simulink model "Marine_LocoMotive_UAV"  (R2018a)
settings: Solver=ode4  StartTime=0.0  StopTime=60  FixedStep=T  RelTol=1e-3
values from neighbouring files (symbols this model uses):
  a_11 = 0.05*m_b    (= 0.625)    [Marine_LocoMotive_UAV_parameters.m]
  a_33 = m_b    (= 12.5)    [Marine_LocoMotive_UAV_parameters.m]
  A_w = 1*1.5/2    (= 0.75)    [Marine_LocoMotive_UAV_parameters.m]
  A_w2 = 1*0.27/2    (= 0.135)    [Marine_LocoMotive_UAV_parameters.m]
  alpha_bar = pi/4    (= 0.785398163397)    [Marine_LocoMotive_UAV_parameters.m]
  Am = sysd.denominator{1}    [Marine_LocoMotive_UAV_parameters.m]
  Am1_LPF = sysd.denominator{1}    [Marine_LocoMotive_UAV_parameters.m]
  Am2_LPF = sysd.denominator{1}    [Marine_LocoMotive_UAV_parameters.m]
  AmAlpha_LPF = sysd.denominator{1}    [Marine_LocoMotive_UAV_parameters.m]
  AmV_LPF = sysd.denominator{1}    [Marine_LocoMotive_UAV_parameters.m]
  AmZ_LPF = sysd.denominator{1}    [Marine_LocoMotive_UAV_parameters.m]
  b_11 = 0    [Marine_LocoMotive_UAV_parameters.m]
  b_33 = 2*m_b*omega_h    (= 27.5578302946)    [Marine_LocoMotive_UAV_parameters.m]
  Bm = sysd.numerator{1}    [Marine_LocoMotive_UAV_parameters.m]
  Bm1_LPF = sysd.numerator{1}    [Marine_LocoMotive_UAV_parameters.m]
  Bm2_LPF = sysd.numerator{1}    [Marine_LocoMotive_UAV_parameters.m]
  BmAlpha_LPF = sysd.numerator{1}    [Marine_LocoMotive_UAV_parameters.m]
  BmV_LPF = sysd.numerator{1}    [Marine_LocoMotive_UAV_parameters.m]
  BmZ_LPF = sysd.numerator{1}    [Marine_LocoMotive_UAV_parameters.m]
  C_S = [5;9]*10^-3    [Marine_LocoMotive_UAV_parameters.m]
  D_x = b_11 + D_s(1)    [Marine_LocoMotive_UAV_parameters.m]
  D_z = b_33 + D_s(2)    [Marine_LocoMotive_UAV_parameters.m]
  dc_M_p = 6.7    [Marine_LocoMotive_UAV_parameters.m]
  Delta_h = (A_im/A_b-0.5)*h_b    (= -0.0625)    [Marine_LocoMotive_UAV_parameters.m]
  epsilon_1 = 5    [Marine_LocoMotive_UAV_parameters.m]
  epsilon_w = 0    [Marine_LocoMotive_UAV_parameters.m]
  epsilon_w2 = pi    (= 3.14159265359)    [Marine_LocoMotive_UAV_parameters.m]
  g = 9.81    [Marine_LocoMotive_UAV_parameters.m]
  gamma_d_p = 2*0.3/0.03*2*0.2*12/4    (= 24)    [Marine_LocoMotive_UAV_parameters.m]
  H = 10    [Marine_LocoMotive_UAV_parameters.m]
  h_b = 0.25    [Marine_LocoMotive_UAV_parameters.m]
  J_a = m_u*Lc_0^2 + (m_u*(Lc_0/2)^2+m_u*Lc_0/12)    (= 111.3)    [Marine_LocoMotive_UAV_parameters.m]
  J_b = m_b*h_b*l_b/12    (= 0.208333333333)    [Marine_LocoMotive_UAV_parameters.m]
  J_u = 0.03    [Marine_LocoMotive_UAV_parameters.m]
  K = 20    [Marine_LocoMotive_UAV_parameters.m]
  k3 = 4.5    [Marine_LocoMotive_UAV_parameters.m]
  k4 = 2    [Marine_LocoMotive_UAV_parameters.m]
  k_w = omega_w^2/g    (= 0.123862835563)    [Marine_LocoMotive_UAV_parameters.m]
  k_w2 = omega_w2^2/g    (= 0.447144836384)    [Marine_LocoMotive_UAV_parameters.m]
  kd_a = 7    [Marine_LocoMotive_UAV_parameters.m]
  kd_t = 6    [Marine_LocoMotive_UAV_parameters.m]
  kd_T = 0.3    [Marine_LocoMotive_UAV_parameters.m]
  kd_x = 5    [Marine_LocoMotive_UAV_parameters.m]
  kd_z = 2    [Marine_LocoMotive_UAV_parameters.m]
  ki_a = 2    [Marine_LocoMotive_UAV_parameters.m]
  ki_T = 0.8    [Marine_LocoMotive_UAV_parameters.m]
  ki_x = 1.2    [Marine_LocoMotive_UAV_parameters.m]
  ki_z = 1    [Marine_LocoMotive_UAV_parameters.m]
  kp_a = 7    [Marine_LocoMotive_UAV_parameters.m]
  kp_t = 10    [Marine_LocoMotive_UAV_parameters.m]
  kp_T = 5    [Marine_LocoMotive_UAV_parameters.m]
  kp_x = 7    [Marine_LocoMotive_UAV_parameters.m]
  kp_z = 3    [Marine_LocoMotive_UAV_parameters.m]
  L = 0.2    [Marine_LocoMotive_UAV_parameters.m]
  l_b = 0.8    [Marine_LocoMotive_UAV_parameters.m]
  Lc_0 = 7    [Marine_LocoMotive_UAV_parameters.m]
  LIMIT_CMD_PITCH = 45*pi/180    (= 0.785398163397)    [Marine_LocoMotive_UAV_parameters.m]
  LIMIT_uCMD_HEIGHT = 3.5*K    (= 70)    [Marine_LocoMotive_UAV_parameters.m]
  M_a = m_u*Lc_0 + m_c*Lc_0    (= 16.1)    [Marine_LocoMotive_UAV_parameters.m]
  m_b = rho_w*Vol_b/4    (= 12.5)    [Marine_LocoMotive_UAV_parameters.m]
  m_c = 0.5    [Marine_LocoMotive_UAV_parameters.m]
  m_u = 1.8    [Marine_LocoMotive_UAV_parameters.m]
  nu_w = 1.787*10^-6    (= 1.787e-06)    [Marine_LocoMotive_UAV_parameters.m]
  omega_w = 2*pi/T_w    (= 1.10231321179)    [Marine_LocoMotive_UAV_parameters.m]
  omega_w2 = 2*pi/T_w2    (= 2.09439510239)    [Marine_LocoMotive_UAV_parameters.m]
  rho_w = 1000    [Marine_LocoMotive_UAV_parameters.m]
  T = 1/100    (= 0.01)    [Marine_LocoMotive_UAV_parameters.m]
  Theta0 = atan2(V_bar*D_x*cos(alpha_bar_0),V_bar*D_x*sin(alpha_bar_0)+m_u*g*cos(alpha_bar_0))    [Marine_LocoMotive_UAV_parameters.m]
  u_s = w_dir*A_w^2*omega_w*k_w*exp(2*k_w*(-Delta_h/2))    [Marine_LocoMotive_UAV_parameters.m]
  u_s2 = w_dir2*A_w2^2*omega_w2*k_w2*exp(2*k_w2*(-Delta_h/2))    [Marine_LocoMotive_UAV_parameters.m]
  u_t = 0*0.2*1    (= 0)    [Marine_LocoMotive_UAV_parameters.m]
  u_w = 0*0.2    (= 0)    [Marine_LocoMotive_UAV_parameters.m]
  V0_b = [u_t+u_w+u_s+u_s2+v_x_w, v_z_w]    [Marine_LocoMotive_UAV_parameters.m]
  V_bar = 5    [Marine_LocoMotive_UAV_parameters.m]
  Vol_b = A_b*l_b    (= 0.05)    [Marine_LocoMotive_UAV_parameters.m]
  w_dir = 1    [Marine_LocoMotive_UAV_parameters.m]
  w_dir2 = 1    [Marine_LocoMotive_UAV_parameters.m]
  X0_b = [0,H+Zeta_0-Delta_h]    [Marine_LocoMotive_UAV_parameters.m]
  zu_bar = X0_b(2) + Lc_0*sin(alpha_bar_0)    [Marine_LocoMotive_UAV_parameters.m]
undefined symbols (not defined in the file or in its folder): DiscIntNeverNeededParam, k_Da, k_Pa, R_b, Zg
libraries: simulink x30, simulink_extras x3
(part 3 of 3)

== system Marine_LocoMotive_UAV/UAV control/u_alpha1 ==
  note: PID
  alpha : Inport
  Xb_ddot1 : Inport  Port=2
  alpha_ref : Inport  Port=3
  "alpha_dot " : Inport  Port=4
  " alpha" : InportShadow
  Add3 : Sum  Inputs=+--
  Add4 : Sum  Inputs=3
  Discrete Transfer Fcn : DiscreteTransferFcn  Commented=on  Numerator=BmAlpha_LPF  Denominator=AmAlpha_LPF
  Discrete Derivative2 : simulink/Discrete/Discrete Derivative  gainval=1.0  ICPrevScaledInput=alpha_bar/T  OutMin=[]  OutMax=[]  OutDataType=fixdt(1, 16)  OutScaling=2^-10  DoSatur=off
  Discrete-Time Integrator : DiscreteIntegrator  SampleTime=-1  LimitOutput=on  UpperSaturationLimit=1  LowerSaturationLimit=-1  ICPrevOutput=DiscIntNeverNeededParam  ICPrevScaledInput=DiscIntNeverNeededParam
  Gain10 : Gain  Gain=kd_a*2
  Gain12 : Gain  Gain=Lc_0
  Gain15 : Gain  Gain=Lc_0
  Gain4 : Gain  Gain=m_u
  Gain6 : Gain  Gain=g
  Gain8 : Gain  Gain=kp_a
  Gain9 : Gain  Gain=ki_a*2
  IC : InitialCondition  Value=0
  Mux : Mux  Inputs=2
  Mux1 : Mux
  Product2 : Product
  Product4 : Product
  Scope{10..11,17..18,26} (5 alike) : Scope
  Sum1 : Sum  Inputs=|+-
  Sum2 : Sum  Inputs=|+-
  Sum7 : Sum  Inputs=|+-
  Trigonometric Function2 : Trigonometry  Operator=cos
  Trigonometric Function3 : Trigonometry  Operator=sincos
  "alpha " : InportShadow
  pid_fb : Scope
  tuner : Gain  Gain=2
  "ua_fb " : Scope
  very high frequency not useful : Gain
  xb_ddot 1 : Selector  InputPortWidth=2  IndexOptions=Index vector (dialog)  Indices=1  OutputSizes=1
  zb_ddot2 : Selector  InputPortWidth=2  IndexOptions=Index vector (dialog)  Indices=1  OutputSizes=1
  u_a : Outport
  wires:
  Gain12/1 -> tuner/1
  very high frequency not useful/1 -> Add3/2
  Mux1/1 -> pid_fb/1
  alpha/1 -> Trigonometric Function2/1
  "alpha "/1 -> Trigonometric Function3/1
  " alpha"/1 -> Sum2/1
  Mux/1 -> Scope26/1
  Trigonometric Function3/2 -> Product4/2
  Discrete-Time Integrator/1 -> Add4/2, Mux1/2  "i"
  Gain15/1 -> very high frequency not useful/1, Scope11/1
  Trigonometric Function2/1 -> Gain6/1
  Trigonometric Function3/1 -> Product2/2
  Product2/1 -> Sum7/1
  Gain9/1 -> Discrete-Time Integrator/1
  xb_ddot 1/1 -> Product2/1
  Gain10/1 -> Mux/2, Mux/1, Add4/3, Mux1/3  "d"
  Xb_ddot1/1 -> xb_ddot 1/1, zb_ddot2/1
  Discrete Derivative2/1 -> IC/1
  Add3/1 -> Gain4/1
  Gain8/1 -> Add4/1, Mux1/1  "p"
  zb_ddot2/1 -> Product4/1
  Product4/1 -> Sum7/2
  tuner/1 -> Add3/3, "ua_fb "/1
  Gain4/1 -> u_a/1  "u_a"
  "alpha_dot "/1 -> Sum1/1
  Add4/1 -> Gain12/1, Mux1/4  "fb"
  alpha_ref/1 -> Discrete Derivative2/1, Sum2/2, Scope18/1
  Sum1/1 -> Gain10/1
  Sum2/1 -> Gain8/1, Gain9/1
  Sum7/1 -> Gain15/1
  Gain6/1 -> Add3/1, Scope10/1
  IC/1 -> Sum1/2, Scope17/1

== system Marine_LocoMotive_UAV/Quadrotor+buoy/3-DOF equations of motion Earth frame/C_123 ==
  "alpha " : Inport
  alpha_dot : Inport  Port=2
  Constant : Constant  Value=0
  Gain : Gain  Gain=-M_a
  Gain1 : Gain  Gain=-M_a
  Product : Product
  Product1 : Product
  Signal Specification1 : SignalSpecification  Dimensions=3
  Signal Specification2 : SignalSpecification  Dimensions=3
  Signal Specification3 : SignalSpecification  Dimensions=3
  Trigonometric Function : Trigonometry  Operator=sincos
  Vector Concatenate1 : Concatenate  NumInputs=3  Mode=Multidimensional array  ConcatenateDimension=2
  Vector Concatenate2 : Concatenate  NumInputs=3
  Vector Concatenate3 : Concatenate  NumInputs=3
  Vector Concatenate4 : Concatenate  NumInputs=3
  C_123 : Outport
  wires:
  Signal Specification3/1 -> Vector Concatenate1/3
  Signal Specification2/1 -> Vector Concatenate1/2
  Signal Specification1/1 -> Vector Concatenate1/1
  Vector Concatenate1/1 -> C_123/1
  Trigonometric Function/2 -> Gain1/1
  Trigonometric Function/1 -> Gain/1
  "alpha "/1 -> Trigonometric Function/1
  Vector Concatenate4/1 -> Signal Specification2/1
  Vector Concatenate2/1 -> Signal Specification1/1
  Vector Concatenate3/1 -> Signal Specification3/1
  Gain/1 -> Product/1
  Gain1/1 -> Product1/1
  Product1/1 -> Vector Concatenate3/1
  Product/1 -> Vector Concatenate3/2
  alpha_dot/1 -> Product1/2, Product/2
  Constant/1 -> Vector Concatenate3/3, Vector Concatenate4/3, Vector Concatenate4/2, Vector Concatenate4/1, Vector Concatenate2/3, Vector Concatenate2/2, Vector Concatenate2/1

== system Marine_LocoMotive_UAV/Quadrotor+buoy/3-DOF equations of motion Earth frame/D_123 ==
  eta_dot_tilde : Inport
  theta_b : Inport  Port=2
  dh : Inport  Port=3
  Constant6 : Constant  Value=[0 0 0]
  Constant7 : Constant  Value=0
  Scope : Scope
  Scope1 : Scope
  Scope2 : Scope
  Vector Concatenate1 : Concatenate  NumInputs=3  Mode=Multidimensional array  ConcatenateDimension=2
  Vector Concatenate2 : Concatenate  NumInputs=3
  Vector Concatenate3 : Concatenate  NumInputs=3
  Vector Concatenate4 : Concatenate
  Vector Concatenate5 : Concatenate
  Vector Concatenate6 : Concatenate
  Water Daming : Subsystem
  Water Daming1 : Subsystem
  D_123 : Outport
  wires:
  Water Daming/2(D22_I) -> Vector Concatenate3/2, Vector Concatenate5/2
  Constant7/1 -> Vector Concatenate3/3, Vector Concatenate2/3
  Constant6/1 -> Vector Concatenate1/3
  Vector Concatenate2/1 -> Vector Concatenate1/1
  Water Daming/1(D11_I) -> Vector Concatenate4/2, Vector Concatenate2/1
  Vector Concatenate3/1 -> Vector Concatenate1/2
  theta_b/1 -> Water Daming1/1(theta), Water Daming/1(theta_b)
  eta_dot_tilde/1 -> Water Daming/2(eta_dot_tilde)
  dh/1 -> Water Daming/3(dh)
  Vector Concatenate1/1 -> D_123/1
  Vector Concatenate4/1 -> Scope/1
  Water Daming1/1(D11_I) -> Vector Concatenate4/1
  Vector Concatenate5/1 -> Scope1/1
  Water Daming1/2(D22_I) -> Vector Concatenate5/1
  Vector Concatenate6/1 -> Scope2/1
  Water Daming1/3(D12_I) -> Vector Concatenate6/1
  Water Daming/3(D12_I) -> Vector Concatenate3/1, Vector Concatenate6/2, Vector Concatenate2/2

== system Marine_LocoMotive_UAV/Quadrotor+buoy/3-DOF equations of motion Earth frame/FB ==
  Constant1 : Constant  Value=rho_w*g
  F_B : Product
  Out1 : Outport
  wires:
  F_B/1 -> Out1/1
  [Vol_im] -> F_B/1
  Constant1/1 -> F_B/2

== system Marine_LocoMotive_UAV/Quadrotor+buoy/3-DOF equations of motion Earth frame/G1 ==
  Constant3 : Constant  Value=0
  Constant4 : Constant  Value=(m_b)*g
  Vector Concatenate : Concatenate
  G : Outport
  wires:
  Vector Concatenate/1 -> G/1
  Constant3/1 -> Vector Concatenate/1  "u1"
  Constant4/1 -> Vector Concatenate/2  "u2"

== system Marine_LocoMotive_UAV/Quadrotor+buoy/3-DOF equations of motion Earth frame/G123 ==
  alpha : Inport
  Constant3 : Constant  Value=0
  Constant4 : Constant  Value=(m_b+m_u+m_c)*g
  Constant5 : Constant  Value=m_u*g*L
  Product5 : Product  Inputs=**  SaturateOnIntegerOverflow=on  InputSameDT=on  OutDataTypeStr=Inherit: Same as first input
  Trigonometric Function : Trigonometry  Operator=cos
  Vector Concatenate : Concatenate  NumInputs=3
  G : Outport
  wires:
  Constant5/1 -> Product5/1
  Trigonometric Function/1 -> Product5/2
  Product5/1 -> Vector Concatenate/3  "u3"
  Constant4/1 -> Vector Concatenate/2  "u2"
  Constant3/1 -> Vector Concatenate/1  "u1"
  alpha/1 -> Trigonometric Function/1
  Vector Concatenate/1 -> G/1

== system Marine_LocoMotive_UAV/Quadrotor+buoy/3-DOF equations of motion Earth frame/M_12 ==
  theta : Inport
  Bias : Bias
  Bias1 : Bias
  Signal Specification1 : SignalSpecification  Dimensions=2
  Signal Specification2 : SignalSpecification  Dimensions=2
  Vector Concatenate1 : Concatenate  Mode=Multidimensional array  ConcatenateDimension=2
  Vector Concatenate2 : Concatenate
  Vector Concatenate3 : Concatenate
  added mass : Subsystem
  M_12 : Outport
  wires:
  Signal Specification2/1 -> Vector Concatenate1/2
  Signal Specification1/1 -> Vector Concatenate1/1
  Vector Concatenate1/1 -> M_12/1
  Bias1/1 -> Vector Concatenate3/2
  Bias/1 -> Vector Concatenate2/1
  added mass/2(M22_I) -> Bias1/1
  added mass/3(M12_I) -> Vector Concatenate2/2, Vector Concatenate3/1
  Vector Concatenate2/1 -> Signal Specification1/1
  added mass/1(M11_I) -> Bias/1
  Vector Concatenate3/1 -> Signal Specification2/1
  theta/1 -> added mass/1(theta)

== system Marine_LocoMotive_UAV/Quadrotor+buoy/3-DOF equations of motion Earth frame/M_123 ==
  theta : Inport
  alpha : Inport  Port=2
  Bias : Bias  Bias=m_u+m_c
  Bias1 : Bias  Bias=m_u+m_c
  Buoy Inertia : Subsystem
  Constant : Constant  Value=J_a
  Gain : Gain  Gain=-M_a
  Gain1 : Gain  Gain=M_a
  Signal Specification1 : SignalSpecification  Dimensions=3
  Signal Specification2 : SignalSpecification  Dimensions=3
  Signal Specification3 : SignalSpecification  Dimensions=3
  Trigonometric Function : Trigonometry  Operator=sincos
  Vector Concatenate1 : Concatenate  NumInputs=3  Mode=Multidimensional array  ConcatenateDimension=2
  Vector Concatenate2 : Concatenate  NumInputs=3
  Vector Concatenate3 : Concatenate  NumInputs=3
  Vector Concatenate4 : Concatenate  NumInputs=3
  M_123 : Outport
  wires:
  theta/1 -> Buoy Inertia/1(theta)
  Vector Concatenate3/1 -> Signal Specification2/1
  Buoy Inertia/1(M11_I) -> Bias/1
  Vector Concatenate2/1 -> Signal Specification1/1
  Vector Concatenate4/1 -> Signal Specification3/1
  Buoy Inertia/3(M12_I) -> Vector Concatenate2/2, Vector Concatenate3/1
  Gain/1 -> Vector Concatenate2/3, Vector Concatenate4/1
  Buoy Inertia/2(M22_I) -> Bias1/1
  Bias/1 -> Vector Concatenate2/1
  Bias1/1 -> Vector Concatenate3/2
  alpha/1 -> Trigonometric Function/1
  Trigonometric Function/1 -> Gain/1
  Trigonometric Function/2 -> Gain1/1
  Gain1/1 -> Vector Concatenate4/2, Vector Concatenate3/3
  Constant/1 -> Vector Concatenate4/3
  Vector Concatenate1/1 -> M_123/1
  Signal Specification1/1 -> Vector Concatenate1/1
  Signal Specification2/1 -> Vector Concatenate1/2
  Signal Specification3/1 -> Vector Concatenate1/3

== system Marine_LocoMotive_UAV/Quadrotor+buoy/3-DOF equations of motion Earth frame/Tension from Buoy, X direction ==
  alpha : Inport
  M12 : Inport  Port=2
  D12 : Inport  Port=3
  Vr,Wr : Inport  Port=4
  Xb_ddot : Inport  Port=5
  G : Inport  Port=6
  FB : Inport  Port=7
  Add1 : Sum  Inputs=+++-
  Constant : Constant  Value=0
  Math Function : Math  Operator=reciprocal  SaturateOnIntegerOverflow=on
  Math Function1 : Math  Operator=reciprocal  SaturateOnIntegerOverflow=on
  Product1 : Product
  Product2 : Product  Inputs=**  Multiplication=Matrix(*)
  Product3 : Product  Inputs=**  Multiplication=Matrix(*)
  Scope5 : Scope
  Trigonometric Function3 : Trigonometry  Operator=sincos
  Vector Concatenate2 : Concatenate
  Vector Concatenate3 : Concatenate
  T x,z : Outport
  wires:
  alpha/1 -> Trigonometric Function3/1
  M12/1 -> Product2/1
  Vr,Wr/1 -> Product3/2
  D12/1 -> Product3/1
  Xb_ddot/1 -> Product2/2
  G/1 -> Add1/3
  Product2/1 -> Add1/2
  Trigonometric Function3/2 -> Math Function/1
  Trigonometric Function3/1 -> Math Function1/1
  Product3/1 -> Add1/1
  Math Function/1 -> Vector Concatenate2/1
  Math Function1/1 -> Vector Concatenate2/2
  Constant/1 -> Vector Concatenate3/1
  Vector Concatenate3/1 -> Add1/4
  FB/1 -> Vector Concatenate3/2
  Product1/1 -> Scope5/1, T x,z/1
  Vector Concatenate2/1 -> Product1/2
  Add1/1 -> Product1/1

== system Marine_LocoMotive_UAV/Quadrotor+buoy/3-DOF equations of motion Earth frame/Tension from UAV, X and r directions ==
  alpha : Inport
  r_p_ddot : Inport  Port=2
  theta_u : Inport  Port=3
  u1 : Inport  Port=4
  Xb_ddot : Inport  Port=5
  Xu : Inport  Port=6
  Add1 : Sum  Inputs=+-+
  Add2 : Sum  Inputs=---
  Add3 : Sum  Commented=on  Inputs=+-
  Discrete Derivative2 : simulink/Discrete/Discrete Derivative  Commented=on  gainval=1.0  ICPrevScaledInput=L*500  OutMin=[]  OutMax=[]  OutDataType=fixdt(1, 16)  OutScaling=2^-10  DoSatur=off
  Discrete Derivative3 : simulink/Discrete/Discrete Derivative  Commented=on  gainval=1.0  ICPrevScaledInput=0  OutMin=[]  OutMax=[]  OutDataType=fixdt(1, 16)  OutScaling=2^-10  DoSatur=off
  Gain14 : Gain  Commented=on
  Gain15 : Gain  Commented=on  Gain=m_u
  Gain5 : Gain  Gain=m_u
  Gain6 : Gain  Gain=m_u*g
  Product10 : Product  Inputs=**  Multiplication=Matrix(*)
  Product12 : Product  Commented=on
  Product7 : Product
  Product9 : Product  Commented=on  Inputs=*/
  Sum4 : Sum  Inputs=|++
  Trigonometric Function2 : Trigonometry
  Trigonometric Function3 : Trigonometry  Operator=sincos
  Trigonometric Function6 : Trigonometry  Commented=on  Operator=cos
  Trigonometric Function8 : Trigonometry  Commented=on
  Vector Concatenate : Concatenate
  alpha1 : InportShadow
  r : Constant  Commented=on  Value=L
  theta_u1 : InportShadow  Port=3
  u2 : InportShadow  Port=4
  x_ddot1 : Selector  Commented=on  InputPortWidth=2  IndexOptions=Index vector (dialog)  Indices=1  OutputSizes=1
  "T, from r" : Outport
  "T, from x simple" : Outport  Port=2
  wires:
  r/1 -> Discrete Derivative2/1
  r_p_ddot/1 -> Add2/1
  alpha/1 -> Trigonometric Function3/1
  Sum4/1 -> Trigonometric Function2/1
  Xb_ddot/1 -> Product10/1
  [alpha] -> Sum4/1
  u1/1 -> Product7/2
  Discrete Derivative3/1 -> Add2/3
  Add2/1 -> Gain5/1
  Trigonometric Function2/1 -> Product7/1
  Discrete Derivative2/1 -> Discrete Derivative3/1
  Trigonometric Function3/1 -> Gain6/1, Vector Concatenate/2
  Product10/1 -> Add2/2
  Gain5/1 -> Add1/1
  theta_u/1 -> Sum4/2
  Add1/1 -> "T, from r"/1
  Gain6/1 -> Add1/2
  Trigonometric Function3/2 -> Vector Concatenate/1
  Product9/1 -> "T, from x simple"/1
  Add3/1 -> Product9/1
  Gain14/1 -> Add3/1
  Trigonometric Function8/1 -> Product12/1
  u2/1 -> Product12/2
  alpha1/1 -> Trigonometric Function6/1
  Product12/1 -> Gain14/1
  x_ddot1/1 -> Gain15/1
  Trigonometric Function6/1 -> Product9/2
  Xu/1 -> x_ddot1/1
  theta_u1/1 -> Trigonometric Function8/1
  Gain15/1 -> Add3/2
  Vector Concatenate/1 -> Product10/2
  Product7/1 -> Add1/3

== system Marine_LocoMotive_UAV/Quadrotor+buoy/3-DOF equations of motion Earth frame/Xu from acc ==
  In1 : Inport
  In2 : Inport  Port=2
  In3 : Inport  Port=3
  (x,z) : DiscreteIntegrator  Commented=on  InitialCondition=[pos_b_ini + L*[cos(alpha_0) sin(alpha_0)]]  SampleTime=-1  ICPrevOutput=DiscIntNeverNeededParam  ICPrevScaledInput=DiscIntNeverNeededParam
  Demux2 : Demux  Commented=on  Outputs=2
  Demux3 : Demux  Commented=on  Outputs=2
  From21 : From  Commented=on  GotoTag=r_p_ddot
  From25 : From  Commented=on  GotoTag=XZb_ddot
  From54 : From  Commented=on  GotoTag=R_Wp_to_W
  Math Function2 : Math  Commented=on  Operator=transpose  SaturateOnIntegerOverflow=on
  Product2 : Product  Commented=on  Multiplication=Matrix(*)
  Sum : Sum  Commented=on  Inputs=|++
  Vector Concatenate7 : Concatenate  Commented=on
  Vector Concatenate8 : Concatenate  Commented=on
  Vector Concatenate9 : Concatenate  Commented=on
  dot(x,z) : DiscreteIntegrator  Commented=on  InitialCondition=[v_b_ini]  SampleTime=-1  ICPrevOutput=DiscIntNeverNeededParam  ICPrevScaledInput=DiscIntNeverNeededParam
  x u : Scope  Commented=on
  x u1 : Scope  Commented=on
  z u : Scope  Commented=on
  Out1 : Outport
  wires:
  From21/1 -> Product2/2
  Vector Concatenate9/1 -> x u1/1
  In3/1 -> Vector Concatenate9/2
  In2/1 -> Math Function2/1
  Sum/1 -> Vector Concatenate9/1, dot(x,z)/1
  From25/1 -> Sum/1
  Product2/1 -> Sum/2
  Demux3/1 -> Vector Concatenate7/2
  From54/1 -> Product2/1
  dot(x,z)/1 -> (x,z)/1
  Demux2/1 -> Vector Concatenate7/1
  (x,z)/1 -> Demux2/1
  Vector Concatenate8/1 -> z u/1
  Demux2/2 -> Vector Concatenate8/1
  Demux3/2 -> Vector Concatenate8/2
  In1/1 -> Demux3/1
  Vector Concatenate7/1 -> x u/1
  Math Function2/1 -> Out1/1

== system Marine_LocoMotive_UAV/Quadrotor+buoy/3-DOF equations of motion Earth frame/buoyancy ==
  z_b : Inport
  zeta : Inport  Port=2
  Constant : Constant  Commented=on  Value=g*rho_w*l_b*R_b
  Manual Switch : ManualSwitch  CurrentSetting=0
  Product : Product  Commented=on
  Scope1 : Scope  Commented=on
  Scope3 : Scope  Commented=on
  V_im cuboid : Subsystem
  f(z_b,zeta) cylinder : Subsystem  Commented=on
  two connected cylindrical buoys : Gain  Commented=on  Gain=2
  two connected cylindrical buoys1 : Gain  Commented=on  Gain=l_b*R_b
  two connected cylindrical buoys2 : Gain  Commented=on  Gain=2
  V_im : Outport
  wires:
  z_b/1 -> V_im cuboid/2(zb), f(z_b,zeta) cylinder/2(zb)
  zeta/1 -> V_im cuboid/1(zeta), f(z_b,zeta) cylinder/1(zeta)
  Product/1 -> two connected cylindrical buoys/1
  Constant/1 -> Scope1/1, Product/2
  f(z_b,zeta) cylinder/1(Out1) -> two connected cylindrical buoys1/1, Product/1, Scope3/1
  Manual Switch/1 -> V_im/1
  V_im cuboid/1(Vol_im) -> Manual Switch/2
  two connected cylindrical buoys1/1 -> two connected cylindrical buoys2/1
  two connected cylindrical buoys2/1 -> Manual Switch/1

== system Marine_LocoMotive_UAV/Quadrotor+buoy/3-DOF equations of motion Earth frame/quadrotor position ==
  X123 : Inport
  Demux : Demux  Outputs=3
  Gain : Gain  Gain=L
  Gain3 : Gain  Gain=L
  Sum : Sum  Inputs=|++
  Sum1 : Sum  Inputs=|++
  Trigonometric Function : Trigonometry  Operator=sincos
  Vector Concatenate3 : Concatenate
  Xu : Outport
  wires:
  Trigonometric Function/2 -> Gain3/1
  Trigonometric Function/1 -> Gain/1
  Demux/3 -> Trigonometric Function/1  "alpha"
  Sum1/1 -> Vector Concatenate3/2
  Vector Concatenate3/1 -> Xu/1
  Gain3/1 -> Sum/2
  Demux/2 -> Sum1/1  "z_b"
  Gain/1 -> Sum1/2
  Sum/1 -> Vector Concatenate3/1
  X123/1 -> Demux/1
  Demux/1 -> Sum/1  "x_b"

== system Marine_LocoMotive_UAV/Quadrotor+buoy/3-DOF equations of motion Earth frame/rotation matrix R  ==
  angle (rad) : Inport
  Gain : Gain  Gain=-1
  Signal Specification1 : SignalSpecification  Dimensions=2
  Signal Specification2 : SignalSpecification  Dimensions=2
  Trigonometric Function1 : Trigonometry  Operator=sincos
  Vector Concatenate1 : Concatenate  Mode=Multidimensional array  ConcatenateDimension=2
  Vector Concatenate2 : Concatenate
  Vector Concatenate3 : Concatenate
  R : Outport
  wires:
  Signal Specification2/1 -> Vector Concatenate1/2
  Signal Specification1/1 -> Vector Concatenate1/1
  Vector Concatenate1/1 -> R/1
  Vector Concatenate2/1 -> Signal Specification1/1
  Vector Concatenate3/1 -> Signal Specification2/1
  angle (rad)/1 -> Trigonometric Function1/1
  Trigonometric Function1/2 -> Vector Concatenate3/2, Vector Concatenate2/1
  Trigonometric Function1/1 -> Vector Concatenate2/2, Gain/1
  Gain/1 -> Vector Concatenate3/1

== system Marine_LocoMotive_UAV/Quadrotor+buoy/3-DOF equations of motion Earth frame/u123 ==
  u1 : Inport
  theta : Inport  Port=2
  V_im : Inport  Port=3
  alpha : Inport  Port=4
  Constant1 : Constant  Value=rho_w*g
  Constant2 : Constant  Commented=on  Value=Vol_b/2
  F_B : Product
  Gain : Gain  Gain=L
  Product1 : Product  Inputs=**  SaturateOnIntegerOverflow=on  InputSameDT=on  OutDataTypeStr=Inherit: Same as first input
  Product6 : Product  Inputs=**  SaturateOnIntegerOverflow=on  InputSameDT=on  OutDataTypeStr=Inherit: Same as first input
  Product7 : Product  Inputs=**  SaturateOnIntegerOverflow=on  InputSameDT=on  OutDataTypeStr=Inherit: Same as first input
  Scope9 : Scope
  Sum1 : Sum  Inputs=|++  SaturateOnIntegerOverflow=on
  Sum2 : Sum  Inputs=|++  SaturateOnIntegerOverflow=on
  Trigonometric Function1 : Trigonometry  Operator=sincos
  Trigonometric Function2 : Trigonometry  Operator=cos
  Vector Concatenate3 : Concatenate  NumInputs=3
  u2 : InportShadow
  u123 : Outport
  wires:
  Product7/1 -> Sum1/1
  u1/1 -> Product7/2, Product6/1
  Trigonometric Function1/2 -> Product7/1
  Product1/1 -> Vector Concatenate3/3
  Vector Concatenate3/1 -> Scope9/1, u123/1
  Product6/1 -> Vector Concatenate3/1
  Sum1/1 -> Vector Concatenate3/2
  Trigonometric Function1/1 -> Product6/2
  F_B/1 -> Sum1/2
  theta/1 -> Sum2/1, Trigonometric Function1/1
  V_im/1 -> F_B/1
  alpha/1 -> Sum2/2
  Sum2/1 -> Trigonometric Function2/1
  Trigonometric Function2/1 -> Gain/1
  Gain/1 -> Product1/2
  u2/1 -> Product1/1
  Constant1/1 -> F_B/2

== system Marine_LocoMotive_UAV/UAV control/Coupling/Coupling ==
  note: atan({U1.sin_psi-U2.cos_psi}/U3)
      |
      | asin{(U2.sin_psi+U1.cos_psi)/u1}
  U1 : Inport
  U3 : Inport  Port=2
  Add5 : Sum  Inputs=2
  Divide1 : Product  Inputs=*/
  Gain : Gain  Gain=m_u
  Product4 : Product
  Product5 : Product
  Saturation : Saturate  UpperLimit=LIMIT_uCMD_HEIGHT  LowerLimit=m_u*g*0.5
  Scope : Scope
  Scope1 : Scope
  Sqrt1 : Sqrt  SaturateOnIntegerOverflow=on
  Trigonometric Function2 : Trigonometry  Operator=atan
  u1 (N) : Outport
  phi_d (rad) : Outport  Port=2
  wires:
  U1/1 -> Divide1/1, Product4/2, Product4/1
  Divide1/1 -> Trigonometric Function2/1
  Trigonometric Function2/1 -> phi_d (rad)/1
  Product4/1 -> Add5/1, Scope/1
  Sqrt1/1 -> Gain/1
  Product5/1 -> Scope1/1, Add5/2
  Add5/1 -> Sqrt1/1
  U3/1 -> Divide1/2, Product5/1, Product5/2
  Saturation/1 -> u1 (N)/1
  Gain/1 -> Saturation/1

== system Marine_LocoMotive_UAV/UAV control/Coupling/sat ==
  u : Inport
  Fcn1 : Fcn  Expr=LIMIT_CMD_PITCH*tanh(u(1)/LIMIT_CMD_PITCH)
  Manual Switch : ManualSwitch
  Saturation1 : Saturate  UpperLimit=LIMIT_CMD_PITCH  LowerLimit=-LIMIT_CMD_PITCH
  sat(u) : Outport
  wires:
  u/1 -> Fcn1/1, Saturation1/1
  Manual Switch/1 -> sat(u)/1
  Saturation1/1 -> Manual Switch/2
  Fcn1/1 -> Manual Switch/1

== system Marine_LocoMotive_UAV/UAV control/Coupling /sat  ==
  u : Inport
  Fcn1 : Fcn  Expr=LIMIT_CMD_PITCH*tanh(u(1)/LIMIT_CMD_PITCH)
  Manual Switch : ManualSwitch
  Saturation1 : Saturate  UpperLimit=LIMIT_CMD_PITCH  LowerLimit=-LIMIT_CMD_PITCH
  sat(u) : Outport
  wires:
  u/1 -> Fcn1/1, Saturation1/1
  Manual Switch/1 -> sat(u)/1
  Saturation1/1 -> Manual Switch/2
  Fcn1/1 -> Manual Switch/1

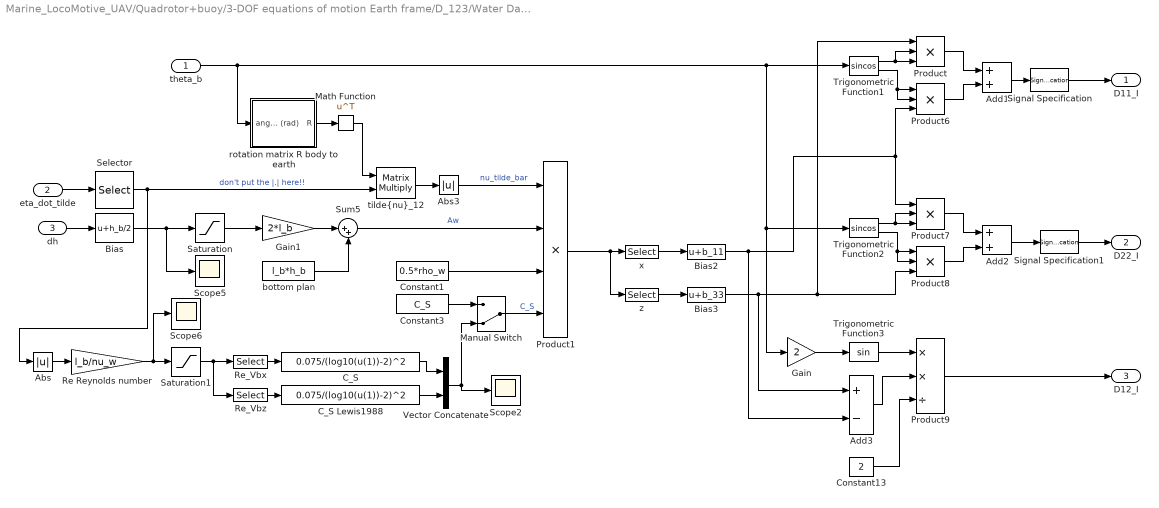
== system Marine_LocoMotive_UAV/Quadrotor+buoy/3-DOF equations of motion Earth frame/D_123/Water Daming ==
  theta_b : Inport
  eta_dot_tilde : Inport  Port=2
  dh : Inport  Port=3
  Abs : Abs
  Abs3 : Abs
  Add1 : Sum
  Add2 : Sum
  Add3 : Sum  Inputs=+-
  Bias : Bias  Bias=h_b/2
  Bias2 : Bias  Bias=b_11
  Bias3 : Bias  Bias=b_33
  C_S : Fcn  Expr=0.075/(log10(u(1))-2)^2
  C_S Lewis1988 : Fcn  Expr=0.075/(log10(u(1))-2)^2
  Constant1 : Constant  Value=0.5*rho_w
  Constant13 : Constant  Value=2
  Constant3 : Constant  Value=C_S
  Gain : Gain  Gain=2
  Gain1 : Gain  Gain=2*l_b
  Manual Switch : ManualSwitch  CurrentSetting=0
  Math Function : Math  Operator=transpose  SaturateOnIntegerOverflow=on
  Product{,6..8} (4 alike) : Product  Inputs=3
  Product1 : Product  Inputs=4
  Product9 : Product  Inputs=**/
  Re Reynolds number : Gain  Gain=l_b/nu_w
  Re_Vbx : Selector  InputPortWidth=2  IndexOptions=Index vector (dialog)  Indices=1  OutputSizes=1
  Re_Vbz : Selector  InputPortWidth=2  IndexOptions=Index vector (dialog)  Indices=2  OutputSizes=1
  Saturation : Saturate  UpperLimit=h_b  LowerLimit=0
  Saturation1 : Saturate  UpperLimit=inf  LowerLimit=0.5*10^5
  Scope2 : Scope
  Scope5 : Scope
  Scope6 : Scope
  Selector : Selector  InputPortWidth=3  IndexOptions=Index vector (dialog)  Indices=[1 2]  OutputSizes=1
  Signal Specification : SignalSpecification  Dimensions=1
  Signal Specification1 : SignalSpecification  Dimensions=1
  Sum5 : Sum  Inputs=|++  SaturateOnIntegerOverflow=on
  Trigonometric Function1 : Trigonometry  Operator=sincos
  Trigonometric Function2 : Trigonometry  Operator=sincos
  Trigonometric Function3 : Trigonometry
  Vector Concatenate : Concatenate
  bottom plan : Constant  Value=l_b*h_b
  rotation matrix R body to earth : Subsystem
  "tilde{nu}_12" : Product  Multiplication=Matrix(*)
  x : Selector  InputPortWidth=2  IndexOptions=Index vector (dialog)  Indices=1  OutputSizes=1
  z : Selector  InputPortWidth=2  IndexOptions=Index vector (dialog)  Indices=1  OutputSizes=1
  D11_I : Outport
  D22_I : Outport  Port=2
  D12_I : Outport  Port=3
  wires:
  Constant13/1 -> Product9/3
  Product7/1 -> Add2/1
  Add3/1 -> Product9/2
  Bias2/1 -> Add3/2, Product7/1, Product6/3
  Bias3/1 -> Add3/1, Product8/3, Product/1
  Product/1 -> Add1/1
  Product6/1 -> Add1/2
  Product8/1 -> Add2/2
  Trigonometric Function1/2 -> Product6/2, Product6/1
  Trigonometric Function2/1 -> Product7/3, Product7/2
  Trigonometric Function2/2 -> Product8/1, Product8/2
  z/1 -> Bias3/1
  Trigonometric Function3/1 -> Product9/1
  Trigonometric Function1/1 -> Product/2, Product/3
  Product9/1 -> D12_I/1
  Gain/1 -> Trigonometric Function3/1
  theta_b/1 -> rotation matrix R body to earth/1(angle (rad)), Gain/1, Trigonometric Function2/1, Trigonometric Function1/1
  rotation matrix R body to earth/1(R) -> Math Function/1
  eta_dot_tilde/1 -> Selector/1
  Math Function/1 -> "tilde{nu}_12"/1
  dh/1 -> Bias/1
  Gain1/1 -> Sum5/1
  bottom plan/1 -> Sum5/2
  Sum5/1 -> Product1/2  "Aw"
  Constant1/1 -> Product1/3
  Manual Switch/1 -> Product1/4  "C_S"
  x/1 -> Bias2/1
  "tilde{nu}_12"/1 -> Abs3/1
  Signal Specification/1 -> D11_I/1
  Add1/1 -> Signal Specification/1
  Add2/1 -> Signal Specification1/1
  Signal Specification1/1 -> D22_I/1
  Product1/1 -> z/1, x/1
  Re Reynolds number/1 -> Scope6/1, Saturation1/1
  Constant3/1 -> Manual Switch/1
  C_S Lewis1988/1 -> Vector Concatenate/2
  C_S/1 -> Vector Concatenate/1
  Bias/1 -> Scope5/1, Saturation/1
  Saturation/1 -> Gain1/1
  Re_Vbx/1 -> C_S/1
  Re_Vbz/1 -> C_S Lewis1988/1
  Saturation1/1 -> Re_Vbz/1, Re_Vbx/1
  Selector/1 -> "tilde{nu}_12"/2, Abs/1  "don't put the |.| here!!"
  Abs3/1 -> Product1/1  "nu_tilde_bar"
  Abs/1 -> Re Reynolds number/1
  Vector Concatenate/1 -> Scope2/1, Manual Switch/2

== system Marine_LocoMotive_UAV/Quadrotor+buoy/3-DOF equations of motion Earth frame/D_123/Water Daming1 ==
  theta : Inport
  Add1 : Sum
  Add2 : Sum
  Add3 : Sum  Inputs=+-
  Constant10 : Constant  Value=D_z
  Constant11 : Constant  Value=D_x
  Constant12 : Constant  Value=D_z
  Constant13 : Constant  Value=2
  Constant7 : Constant  Value=D_x
  Constant8 : Constant  Value=D_z
  Constant9 : Constant  Value=D_x
  Gain : Gain  Gain=2
  Product{,6..8} (4 alike) : Product  Inputs=3
  Product9 : Product  Inputs=**/
  Trigonometric Function1 : Trigonometry  Operator=sincos
  Trigonometric Function2 : Trigonometry  Operator=sincos
  Trigonometric Function3 : Trigonometry
  D11_I : Outport
  D22_I : Outport  Port=2
  D12_I : Outport  Port=3
  wires:
  Gain/1 -> Trigonometric Function3/1
  Add1/1 -> D11_I/1
  Product9/1 -> D12_I/1
  theta/1 -> Trigonometric Function1/1, Trigonometric Function2/1, Gain/1
  Trigonometric Function1/1 -> Product/3, Product/2
  Trigonometric Function3/1 -> Product9/1
  Constant8/1 -> Product/1
  Trigonometric Function2/2 -> Product8/2, Product8/1
  Trigonometric Function2/1 -> Product7/2, Product7/3
  Trigonometric Function1/2 -> Product6/1, Product6/2
  Product8/1 -> Add2/2
  Add2/1 -> D22_I/1
  Product6/1 -> Add1/2
  Product/1 -> Add1/1
  Constant10/1 -> Product8/3
  Constant12/1 -> Add3/1
  Constant7/1 -> Product6/3
  Constant11/1 -> Add3/2
  Add3/1 -> Product9/2
  Product7/1 -> Add2/1
  Constant13/1 -> Product9/3
  Constant9/1 -> Product7/1

== system Marine_LocoMotive_UAV/Quadrotor+buoy/3-DOF equations of motion Earth frame/M_12/added mass ==
  theta : Inport
  Add1 : Sum
  Add2 : Sum
  Add3 : Sum  Inputs=+-
  Constant13 : Constant  Value=2
  Gain : Gain  Gain=2
  M11 : Constant  Value=m_b+a_ii(1)
  "M11 " : Constant  Value=m_b+a_ii(1)
  M11 1 : Constant  Value=m_b+a_ii(1)
  "M22 " : Constant  Value=m_b+a_ii(2)
  M22 1 : Constant  Value=m_b+a_ii(2)
  M_22 : Constant  Value=m_b+a_ii(2)
  Product{,6..8} (4 alike) : Product  Inputs=3
  Product9 : Product  Inputs=**/
  Trigonometric Function1 : Trigonometry  Operator=sincos
  Trigonometric Function2 : Trigonometry  Operator=sincos
  Trigonometric Function3 : Trigonometry
  M11_I : Outport
  M22_I : Outport  Port=2
  M12_I : Outport  Port=3
  wires:
  Gain/1 -> Trigonometric Function3/1
  "M11 "/1 -> Product7/1
  Constant13/1 -> Product9/3
  Product7/1 -> Add2/1
  Add3/1 -> Product9/2
  M11 1/1 -> Add3/2
  M11/1 -> Product6/3
  M22 1/1 -> Add3/1
  "M22 "/1 -> Product8/3
  Product/1 -> Add1/1
  Product6/1 -> Add1/2
  Add2/1 -> M22_I/1
  Product8/1 -> Add2/2
  Trigonometric Function1/2 -> Product6/2, Product6/1
  Trigonometric Function2/1 -> Product7/3, Product7/2
  Trigonometric Function2/2 -> Product8/1, Product8/2
  M_22/1 -> Product/1
  Trigonometric Function3/1 -> Product9/1
  Trigonometric Function1/1 -> Product/2, Product/3
  theta/1 -> Gain/1, Trigonometric Function2/1, Trigonometric Function1/1
  Product9/1 -> M12_I/1
  Add1/1 -> M11_I/1

== system Marine_LocoMotive_UAV/Quadrotor+buoy/3-DOF equations of motion Earth frame/M_123/Buoy Inertia ==
  theta : Inport
  Add1 : Sum
  Add2 : Sum
  Add3 : Sum  Inputs=+-
  Constant13 : Constant  Value=2
  Gain : Gain  Gain=2
  M11 : Constant  Value=m_b+a_ii(1)
  "M11 " : Constant  Value=m_b+a_ii(1)
  M11 1 : Constant  Value=m_b+a_ii(1)
  "M22 " : Constant  Value=m_b+a_ii(2)
  M22 1 : Constant  Value=m_b+a_ii(2)
  M_22 : Constant  Value=m_b+a_ii(2)
  Product{,6..8} (4 alike) : Product  Inputs=3
  Product9 : Product  Inputs=**/
  Trigonometric Function1 : Trigonometry  Operator=sincos
  Trigonometric Function2 : Trigonometry  Operator=sincos
  Trigonometric Function3 : Trigonometry
  M11_I : Outport
  M22_I : Outport  Port=2
  M12_I : Outport  Port=3
  wires:
  Add1/1 -> M11_I/1
  Product9/1 -> M12_I/1
  theta/1 -> Trigonometric Function1/1, Trigonometric Function2/1, Gain/1
  Trigonometric Function1/1 -> Product/3, Product/2
  Trigonometric Function3/1 -> Product9/1
  M_22/1 -> Product/1
  Trigonometric Function2/2 -> Product8/2, Product8/1
  Trigonometric Function2/1 -> Product7/2, Product7/3
  Trigonometric Function1/2 -> Product6/1, Product6/2
  Product8/1 -> Add2/2
  Add2/1 -> M22_I/1
  Product6/1 -> Add1/2
  Product/1 -> Add1/1
  "M22 "/1 -> Product8/3
  M22 1/1 -> Add3/1
  M11/1 -> Product6/3
  M11 1/1 -> Add3/2
  Add3/1 -> Product9/2
  Product7/1 -> Add2/1
  Constant13/1 -> Product9/3
  "M11 "/1 -> Product7/1
  Gain/1 -> Trigonometric Function3/1

== system Marine_LocoMotive_UAV/Quadrotor+buoy/3-DOF equations of motion Earth frame/buoyancy/V_im cuboid ==
  zeta : Inport
  zb : Inport  Port=2
  Constant : Constant  Value=l_b*h_b
  Product3 : Product  SaturateOnIntegerOverflow=on  InputSameDT=on  OutDataTypeStr=Inherit: Same as first input
  Saturation : Saturate  UpperLimit=h_b/2  LowerLimit=-h_b/2
  Scope4 : Scope
  Sum : Sum  Inputs=|++
  Sum2 : Sum  Inputs=|+-  SaturateOnIntegerOverflow=on
  Vol_b/2 : Constant  Value=l_b*h_b*h_b/2
  Vol_im : Outport
  wires:
  Saturation/1 -> Product3/1
  Sum2/1 -> Saturation/1, Scope4/1  "d"
  Product3/1 -> Sum/1
  Constant/1 -> Product3/2
  Sum/1 -> Vol_im/1
  Vol_b/2/1 -> Sum/2
  zeta/1 -> Sum2/1
  zb/1 -> Sum2/2

== system Marine_LocoMotive_UAV/Quadrotor+buoy/3-DOF equations of motion Earth frame/buoyancy/f(z_b,zeta) cylinder ==
  note: This model is valid for d<=R
  zeta : Inport
  zb : Inport  Port=2
  Bias : Bias  Bias=1
  Constant : Constant  Value=R_b
  Product3 : Product  Inputs=*/  SaturateOnIntegerOverflow=on  InputSameDT=on  OutDataTypeStr=Inherit: Same as first input
  Product4 : Product  SaturateOnIntegerOverflow=on  InputSameDT=on  OutDataTypeStr=Inherit: Same as first input
  Product5 : Product  SaturateOnIntegerOverflow=on  InputSameDT=on  OutDataTypeStr=Inherit: Same as first input
  Product6 : Product  SaturateOnIntegerOverflow=on  InputSameDT=on  OutDataTypeStr=Inherit: Same as first input
  Saturation : Saturate  UpperLimit=R_b  LowerLimit=0
  Scope{1..4} (4 alike) : Scope
  Sqrt : Sqrt  SaturateOnIntegerOverflow=on
  Sum2 : Sum  Inputs=-+|  SaturateOnIntegerOverflow=on
  Sum3 : Sum  Inputs=-+|  SaturateOnIntegerOverflow=on
  Unary Minus : UnaryMinus
  acos : Trigonometry  Operator=acos
  Out1 : Outport
  wires:
  Constant/1 -> Product5/2, Product3/2
  Bias/1 -> Sqrt/1
  Product5/1 -> Scope1/1, Sum3/2
  Product4/1 -> Sum3/1
  Product6/1 -> Unary Minus/1
  Unary Minus/1 -> Bias/1
  Sum2/1 -> Scope4/1, Saturation/1  "d"
  Product3/1 -> acos/1, Product6/2, Product6/1
  Sqrt/1 -> Product4/1, Scope3/1
  acos/1 -> Product5/1
  zb/1 -> Sum2/2
  zeta/1 -> Sum2/1
  Sum3/1 -> Out1/1
  Saturation/1 -> Scope2/1, Product4/2, Product3/1

== system Marine_LocoMotive_UAV/Quadrotor+buoy/3-DOF equations of motion Earth frame/D_123/Water Daming/rotation matrix R body to earth ==
  angle (rad) : Inport
  Gain : Gain  Gain=-1
  Signal Specification1 : SignalSpecification  Dimensions=2
  Signal Specification2 : SignalSpecification  Dimensions=2
  Trigonometric Function1 : Trigonometry  Operator=sincos
  Vector Concatenate1 : Concatenate  Mode=Multidimensional array  ConcatenateDimension=2
  Vector Concatenate2 : Concatenate
  Vector Concatenate3 : Concatenate
  R : Outport
  wires:
  Gain/1 -> Vector Concatenate3/1
  Trigonometric Function1/1 -> Gain/1, Vector Concatenate2/2
  Trigonometric Function1/2 -> Vector Concatenate2/1, Vector Concatenate3/2
  angle (rad)/1 -> Trigonometric Function1/1
  Vector Concatenate3/1 -> Signal Specification2/1
  Vector Concatenate2/1 -> Signal Specification1/1
  Vector Concatenate1/1 -> R/1
  Signal Specification1/1 -> Vector Concatenate1/1
  Signal Specification2/1 -> Vector Concatenate1/2
